simulink model "Discomfort"  (R2023b)
settings: Solver=VariableStepAuto  StartTime=0.0  StopTime=10  RelTol=1e-3
values from neighbouring files (symbols this model uses):
  a = 1.35    [Parameters.m]
  b = 1.5    [Parameters.m]
  d = 3    [Parameters.m]
  g = 9.81    [Parameters.m]
  I = 650    [Parameters.m]
  Kt = 14e4    (= 140000)    [Parameters.m]
  L = 3.7    [Parameters.m]
  Mw = 20    [Parameters.m]
  v = [1, 2, 3, 5, 8, 10]    [Parameters.m]
libraries: CarModelLibrary x9, simulink x6, SpeedBumpLibrary x4, spsRMSLib x3
settings Model: Creator=fb552  LastModifiedBy=Francesco
settings SolverCC: AlgebraicLoopSolver=TrustRegion
settings DataIOCC: ReturnWorkspaceOutputsName=SDOSimTest_Log
settings DebuggingCC: UnconnectedInputMsg=warning  UnconnectedOutputMsg=warning  UnconnectedLineMsg=warning
settings ModelReferenceCC: EnableRefExpFcnMdlSchedulingChecks=on

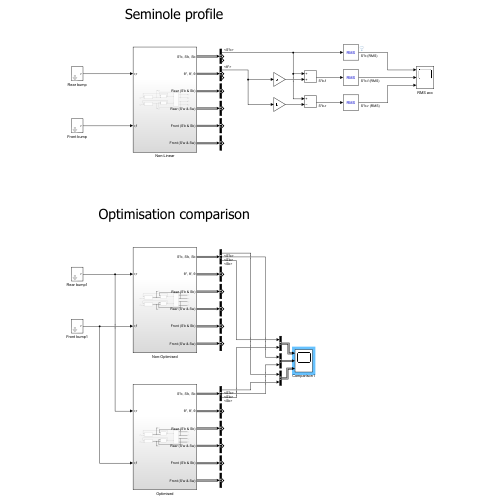
[thumbnail: Simulink's stored preview of the top-level diagram]
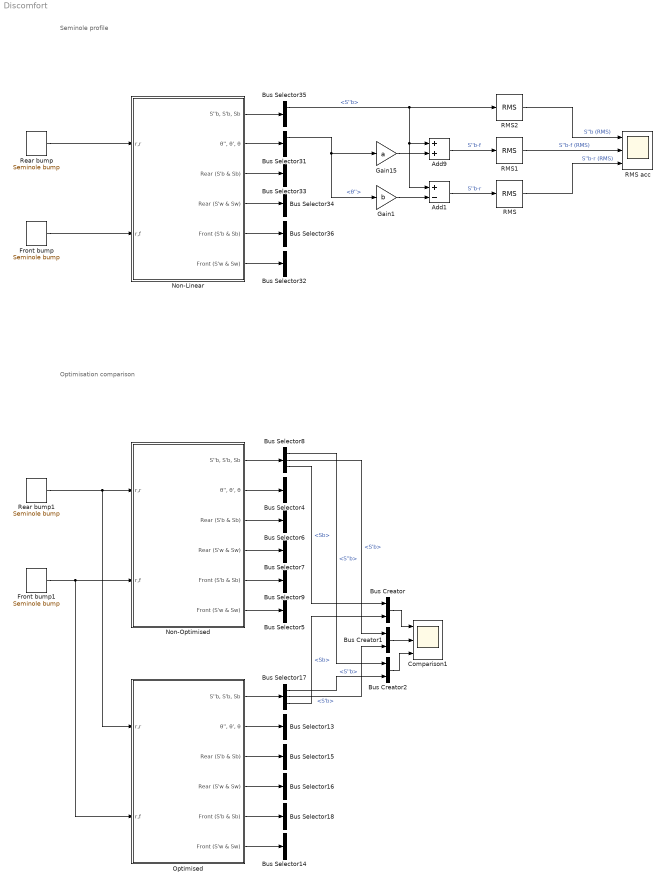
== system Discomfort ==
  note: Seminole profile
  note: Optimisation comparison
  Add1 : Sum  Inputs=+-
  Add9 : Sum
  Bus Creator : BusCreator  Inputs=2
  Bus Creator1 : BusCreator  Inputs=2
  Bus Creator2 : BusCreator  Inputs=2
  Bus Selector13 : BusSelector  OutputSignals=θ
  Bus Selector{5,7,14,16,32,34} (6 alike) : BusSelector  OutputSignals=Sw
  Bus Selector{6,9,15,18,33,36} (6 alike) : BusSelector  OutputSignals=Sb
  Bus Selector17 : BusSelector  OutputSignals=S''b,S'b,Sb
  Bus Selector31 : BusSelector  OutputSignals=θ'',θ',θ
  Bus Selector35 : BusSelector  OutputSignals=S''b,S'b,Sb
  Bus Selector4 : BusSelector  OutputSignals=θ
  Bus Selector8 : BusSelector  OutputSignals=S''b,S'b,Sb
  Comparison1 : Scope  NumInputPorts=3
  Front bump : SpeedBumpLibrary/Seminole bump  h=h  d=d  L=L+d  v=v(5)  delta=0  n=5
  Front bump1 : SpeedBumpLibrary/Seminole bump  h=h  d=d  L=L+d  v=v(5)  delta=0  n=5
  Gain1 : Gain  Gain=b
  Gain15 : Gain  Gain=a
  Non-Linear : Subsystem
  Non-Optimised : Subsystem
  Optimised : Subsystem
  RMS : spsRMSLib/RMS  TrueRMS=on  Freq=60  RMSInit=120  Ts=0
  RMS acc : Scope  NumInputPorts=3
  RMS1 : spsRMSLib/RMS  TrueRMS=on  Freq=60  RMSInit=120  Ts=0
  RMS2 : spsRMSLib/RMS  TrueRMS=on  Freq=60  RMSInit=120  Ts=0
  Rear bump : SpeedBumpLibrary/Seminole bump  h=h  d=d  L=L+d  v=v(5)  delta=a+b  n=5
  Rear bump1 : SpeedBumpLibrary/Seminole bump  h=h  d=d  L=L+d  v=v(5)  delta=a+b  n=5
  wires:
  Non-Linear/2("θ'', θ', θ") -> Bus Selector31/1
  Non-Linear/6(Front (S'w & Sw)) -> Bus Selector32/1
  Non-Linear/4(Rear (S'w & Sw)) -> Bus Selector34/1
  Non-Linear/5(Front (S'b & Sb)) -> Bus Selector36/1
  Non-Linear/1("S''b, S'b, Sb") -> Bus Selector35/1
  Non-Linear/3(Rear (S'b & Sb)) -> Bus Selector33/1
  Gain15/1 -> Add9/2
  Gain1/1 -> Add1/2
  Bus Selector35/1 -> Add1/1, Add9/1, RMS2/1  "<S''b>"
  Bus Selector31/1 -> Gain1/1, Gain15/1  "<θ''>"
  Add1/1 -> RMS/1  "S''b-r"
  Add9/1 -> RMS1/1  "S''b-f"
  RMS1/1 -> RMS acc/2  "S''b-f (RMS)"
  RMS2/1 -> RMS acc/1  "S''b (RMS)"
  RMS/1 -> RMS acc/3  "S''b-r (RMS)"
  Non-Optimised/1("S''b, S'b, Sb") -> Bus Selector8/1
  Non-Optimised/3(Rear (S'b & Sb)) -> Bus Selector6/1
  Non-Optimised/5(Front (S'b & Sb)) -> Bus Selector9/1
  Non-Optimised/2("θ'', θ', θ") -> Bus Selector4/1
  Non-Optimised/4(Rear (S'w & Sw)) -> Bus Selector7/1
  Non-Optimised/6(Front (S'w & Sw)) -> Bus Selector5/1
  Optimised/6(Front (S'w & Sw)) -> Bus Selector14/1
  Optimised/4(Rear (S'w & Sw)) -> Bus Selector16/1
  Optimised/3(Rear (S'b & Sb)) -> Bus Selector15/1
  Optimised/5(Front (S'b & Sb)) -> Bus Selector18/1
  Optimised/2("θ'', θ', θ") -> Bus Selector13/1
  Front bump1/1 -> Optimised/2(r,f), Non-Optimised/2(r,f)
  Rear bump1/1 -> Optimised/1(r,r), Non-Optimised/1(r,r)
  Optimised/1("S''b, S'b, Sb") -> Bus Selector17/1
  Rear bump/1 -> Non-Linear/1(r,r)
  Front bump/1 -> Non-Linear/2(r,f)
  Bus Creator2/1 -> Comparison1/3
  Bus Creator1/1 -> Comparison1/2
  Bus Creator/1 -> Comparison1/1
  Bus Selector17/1 -> Bus Creator2/2  "<S''b>"
  Bus Selector8/1 -> Bus Creator2/1  "<S''b>"
  Bus Selector8/2 -> Bus Creator1/1  "<S'b>"
  Bus Selector17/2 -> Bus Creator1/2  "<S'b>"
  Bus Selector17/3 -> Bus Creator/2  "<Sb>"
  Bus Selector8/3 -> Bus Creator/1  "<Sb>"

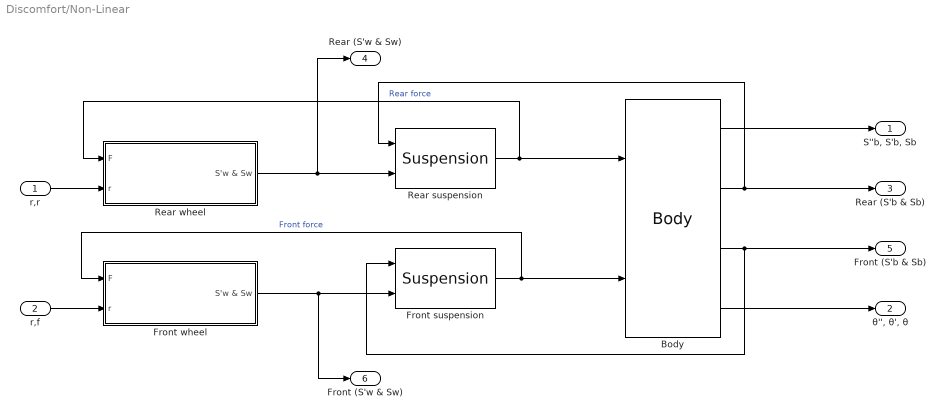
== system Discomfort/Non-Linear ==
  r,r : Inport
  r,f : Inport  Port=2
  Body : CarModelLibrary/Body  mb=Mb  I=I  a=a  b=b
  Front suspension : CarModelLibrary/Suspension  ks=Ks  ksstiff=Kstiff  x0=x0  csb=Csc  csr=Cse
  Front wheel : Subsystem  AncestorBlock=CarModelLibrary/Wheel  mask{mw=Mw, Kt=Kt, g=g}
      mask prompts: mw "Wheel Mass (Kg)"; Kt "Tyre Stiffness"; g "Gravitational acceleration"
  Rear suspension : CarModelLibrary/Suspension  ks=Ks  ksstiff=Kstiff  x0=x0  csb=Csc  csr=Cse
  Rear wheel : Subsystem  AncestorBlock=CarModelLibrary/Wheel  mask{mw=Mw, Kt=Kt, g=g}
      mask prompts: mw "Wheel Mass (Kg)"; Kt "Tyre Stiffness"; g "Gravitational acceleration"
  "S''b, S'b, Sb" : Outport
  "θ'', θ', θ" : Outport  Port=2
  Rear (S'b & Sb) : Outport  Port=3
  Rear (S'w & Sw) : Outport  Port=4
  Front (S'b & Sb) : Outport  Port=5
  Front (S'w & Sw) : Outport  Port=6
  wires:
  Body/1 -> "S''b, S'b, Sb"/1
  Body/2 -> Rear suspension/1, Rear (S'b & Sb)/1
  Front wheel/1(S'w & Sw) -> Front suspension/2, Front (S'w & Sw)/1
  Rear wheel/1(S'w & Sw) -> Rear suspension/2, Rear (S'w & Sw)/1
  Body/4 -> "θ'', θ', θ"/1
  Body/3 -> Front suspension/1, Front (S'b & Sb)/1
  Rear suspension/1 -> Body/1, Rear wheel/1(F)  "Rear force"
  r,r/1 -> Rear wheel/2(r)
  r,f/1 -> Front wheel/2(r)
  Front suspension/1 -> Front wheel/1(F), Body/2  "Front force"

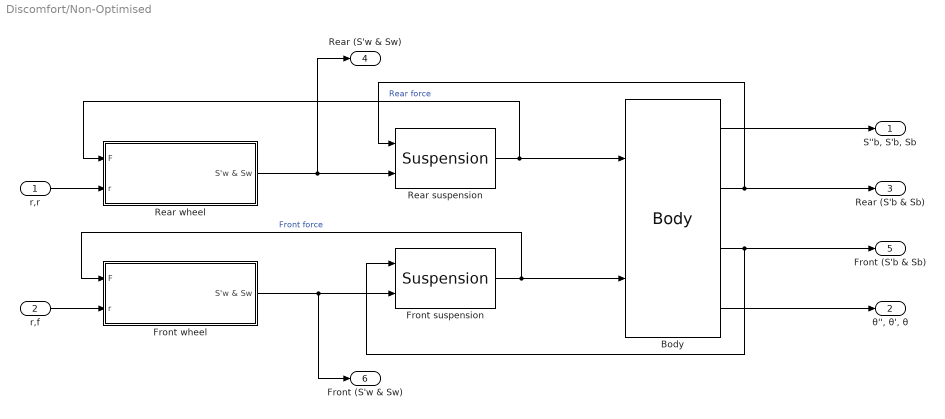
== system Discomfort/Non-Optimised ==
  r,r : Inport
  r,f : Inport  Port=2
  Body : CarModelLibrary/Body  mb=Mb  I=I  a=a  b=b
  Front suspension : CarModelLibrary/Suspension  ks=2e4  ksstiff=20  x0=x0  csb=600  csr=1200
  Front wheel : Subsystem  AncestorBlock=CarModelLibrary/Wheel  mask{mw=Mw, Kt=Kt, g=g}
      mask prompts: mw "Wheel Mass (Kg)"; Kt "Tyre Stiffness"; g "Gravitational acceleration"
  Rear suspension : CarModelLibrary/Suspension  ks=2e4  ksstiff=20  x0=x0  csb=600  csr=1200
  Rear wheel : Subsystem  AncestorBlock=CarModelLibrary/Wheel  mask{mw=Mw, Kt=Kt, g=g}
      mask prompts: mw "Wheel Mass (Kg)"; Kt "Tyre Stiffness"; g "Gravitational acceleration"
  "S''b, S'b, Sb" : Outport
  "θ'', θ', θ" : Outport  Port=2
  Rear (S'b & Sb) : Outport  Port=3
  Rear (S'w & Sw) : Outport  Port=4
  Front (S'b & Sb) : Outport  Port=5
  Front (S'w & Sw) : Outport  Port=6
  wires:
  Body/1 -> "S''b, S'b, Sb"/1
  Body/2 -> Rear suspension/1, Rear (S'b & Sb)/1
  Front wheel/1(S'w & Sw) -> Front suspension/2, Front (S'w & Sw)/1
  Rear wheel/1(S'w & Sw) -> Rear suspension/2, Rear (S'w & Sw)/1
  Body/4 -> "θ'', θ', θ"/1
  Body/3 -> Front suspension/1, Front (S'b & Sb)/1
  Rear suspension/1 -> Body/1, Rear wheel/1(F)  "Rear force"
  r,r/1 -> Rear wheel/2(r)
  r,f/1 -> Front wheel/2(r)
  Front suspension/1 -> Front wheel/1(F), Body/2  "Front force"

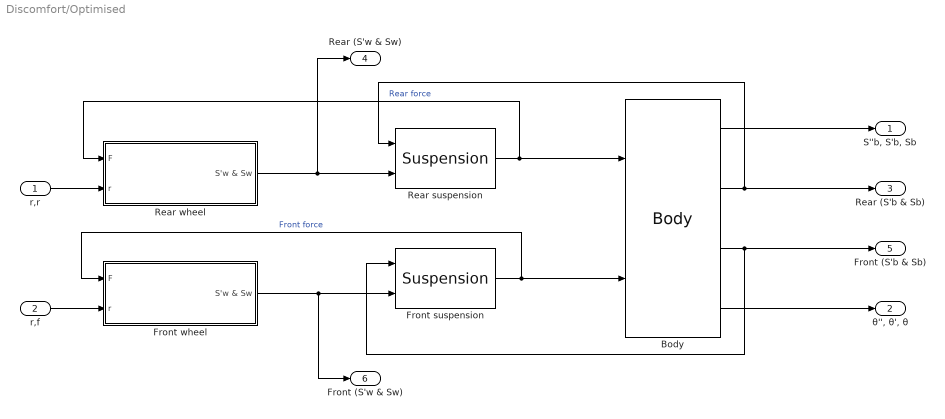
== system Discomfort/Optimised ==
  r,r : Inport
  r,f : Inport  Port=2
  Body : CarModelLibrary/Body  mb=Mb  I=I  a=a  b=b
  Front suspension : CarModelLibrary/Suspension  ks=Ks  ksstiff=Kstiff  x0=x0  csb=Csc  csr=Cse
  Front wheel : Subsystem  AncestorBlock=CarModelLibrary/Wheel  mask{mw=Mw, Kt=Kt, g=g}
      mask prompts: mw "Wheel Mass (Kg)"; Kt "Tyre Stiffness"; g "Gravitational acceleration"
  Rear suspension : CarModelLibrary/Suspension  ks=Ks  ksstiff=Kstiff  x0=x0  csb=Csc  csr=Cse
  Rear wheel : Subsystem  AncestorBlock=CarModelLibrary/Wheel  mask{mw=Mw, Kt=Kt, g=g}
      mask prompts: mw "Wheel Mass (Kg)"; Kt "Tyre Stiffness"; g "Gravitational acceleration"
  "S''b, S'b, Sb" : Outport
  "θ'', θ', θ" : Outport  Port=2
  Rear (S'b & Sb) : Outport  Port=3
  Rear (S'w & Sw) : Outport  Port=4
  Front (S'b & Sb) : Outport  Port=5
  Front (S'w & Sw) : Outport  Port=6
  wires:
  Body/1 -> "S''b, S'b, Sb"/1
  Body/2 -> Rear suspension/1, Rear (S'b & Sb)/1
  Front wheel/1(S'w & Sw) -> Front suspension/2, Front (S'w & Sw)/1
  Rear wheel/1(S'w & Sw) -> Rear suspension/2, Rear (S'w & Sw)/1
  Body/4 -> "θ'', θ', θ"/1
  Body/3 -> Front suspension/1, Front (S'b & Sb)/1
  Rear suspension/1 -> Body/1, Rear wheel/1(F)  "Rear force"
  r,r/1 -> Rear wheel/2(r)
  r,f/1 -> Front wheel/2(r)
  Front suspension/1 -> Front wheel/1(F), Body/2  "Front force"

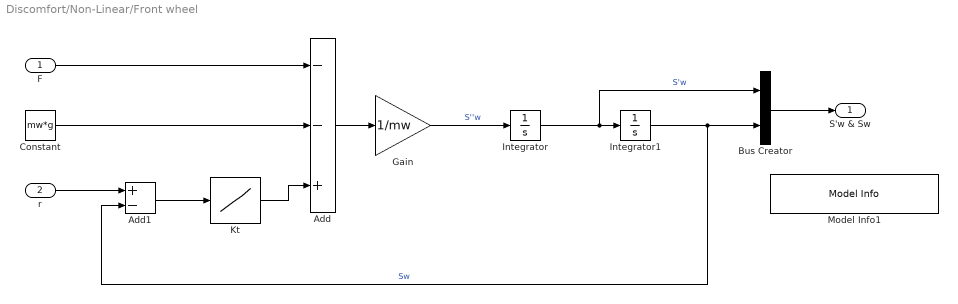
== system Discomfort/Non-Linear/Front wheel ==
  F : Inport
  r : Inport  Port=2
  Add : Sum  Inputs=--+
  Add1 : Sum  Inputs=+-
  Bus Creator : BusCreator  Inputs=2
  Constant : Constant  Value=mw*g
  Gain : Gain  Gain=1/mw
  Integrator : Integrator
  Integrator1 : Integrator
  Kt : Lookup_n-D  NumberOfTableDimensions=1  BreakpointsForDimension1=[-1, 0, 1]  Table=[0, 0, Kt]  InternalRulePriority=Speed  RndMeth=Simplest
  Model Info1 : simulink/Model-Wide Utilities/Model Info  Frame=on  DisplayStringWithTags=m * S''w = -F + Kt (r-S) - m*g  HorizontalTextAlignment=Center  LeftAlignmentValue=0.5
  S'w & Sw : Outport
  wires:
  Kt/1 -> Add/3
  F/1 -> Add/1
  Constant/1 -> Add/2
  Gain/1 -> Integrator/1  "S''w"
  Add/1 -> Gain/1
  Integrator1/1 -> Add1/2, Bus Creator/2  "Sw"
  Bus Creator/1 -> S'w & Sw/1
  Integrator/1 -> Integrator1/1, Bus Creator/1  "S'w"
  Add1/1 -> Kt/1
  r/1 -> Add1/1

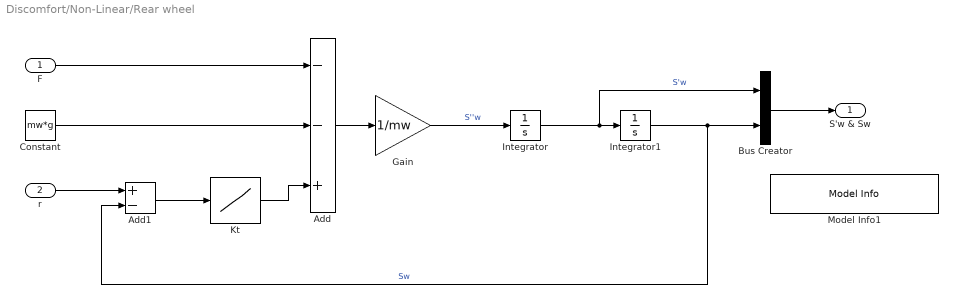
== system Discomfort/Non-Linear/Rear wheel ==
  F : Inport
  r : Inport  Port=2
  Add : Sum  Inputs=--+
  Add1 : Sum  Inputs=+-
  Bus Creator : BusCreator  Inputs=2
  Constant : Constant  Value=mw*g
  Gain : Gain  Gain=1/mw
  Integrator : Integrator
  Integrator1 : Integrator
  Kt : Lookup_n-D  NumberOfTableDimensions=1  BreakpointsForDimension1=[-1, 0, 1]  Table=[0, 0, Kt]  InternalRulePriority=Speed  RndMeth=Simplest
  Model Info1 : simulink/Model-Wide Utilities/Model Info  Frame=on  DisplayStringWithTags=m * S''w = -F + Kt (r-S) - m*g  HorizontalTextAlignment=Center  LeftAlignmentValue=0.5
  S'w & Sw : Outport
  wires:
  Kt/1 -> Add/3
  F/1 -> Add/1
  Constant/1 -> Add/2
  Gain/1 -> Integrator/1  "S''w"
  Add/1 -> Gain/1
  Integrator1/1 -> Add1/2, Bus Creator/2  "Sw"
  Bus Creator/1 -> S'w & Sw/1
  Integrator/1 -> Integrator1/1, Bus Creator/1  "S'w"
  Add1/1 -> Kt/1
  r/1 -> Add1/1

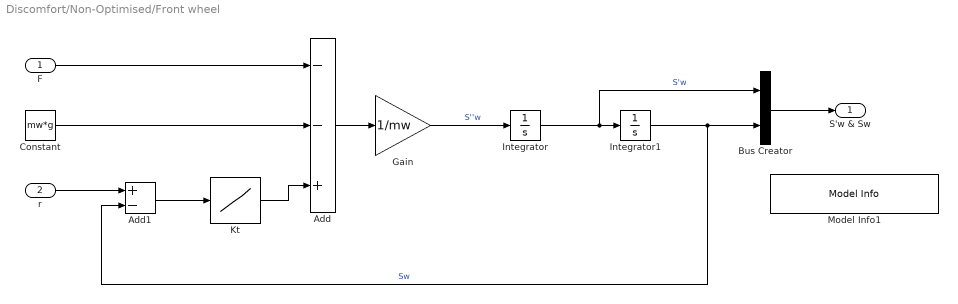
== system Discomfort/Non-Optimised/Front wheel ==
  F : Inport
  r : Inport  Port=2
  Add : Sum  Inputs=--+
  Add1 : Sum  Inputs=+-
  Bus Creator : BusCreator  Inputs=2
  Constant : Constant  Value=mw*g
  Gain : Gain  Gain=1/mw
  Integrator : Integrator
  Integrator1 : Integrator
  Kt : Lookup_n-D  NumberOfTableDimensions=1  BreakpointsForDimension1=[-1, 0, 1]  Table=[0, 0, Kt]  InternalRulePriority=Speed  RndMeth=Simplest
  Model Info1 : simulink/Model-Wide Utilities/Model Info  Frame=on  DisplayStringWithTags=m * S''w = -F + Kt (r-S) - m*g  HorizontalTextAlignment=Center  LeftAlignmentValue=0.5
  S'w & Sw : Outport
  wires:
  Kt/1 -> Add/3
  F/1 -> Add/1
  Constant/1 -> Add/2
  Gain/1 -> Integrator/1  "S''w"
  Add/1 -> Gain/1
  Integrator1/1 -> Add1/2, Bus Creator/2  "Sw"
  Bus Creator/1 -> S'w & Sw/1
  Integrator/1 -> Integrator1/1, Bus Creator/1  "S'w"
  Add1/1 -> Kt/1
  r/1 -> Add1/1

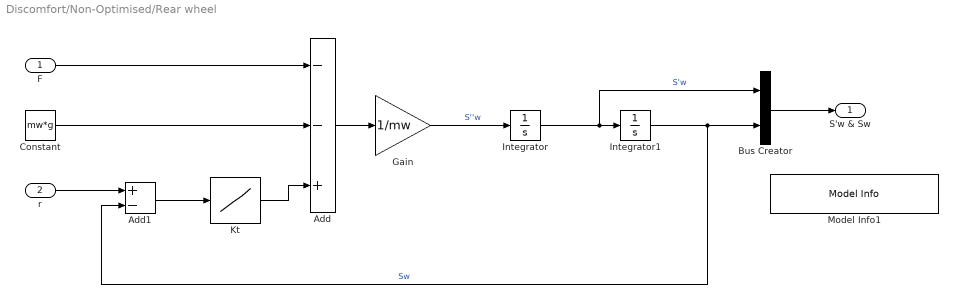
== system Discomfort/Non-Optimised/Rear wheel ==
  F : Inport
  r : Inport  Port=2
  Add : Sum  Inputs=--+
  Add1 : Sum  Inputs=+-
  Bus Creator : BusCreator  Inputs=2
  Constant : Constant  Value=mw*g
  Gain : Gain  Gain=1/mw
  Integrator : Integrator
  Integrator1 : Integrator
  Kt : Lookup_n-D  NumberOfTableDimensions=1  BreakpointsForDimension1=[-1, 0, 1]  Table=[0, 0, Kt]  InternalRulePriority=Speed  RndMeth=Simplest
  Model Info1 : simulink/Model-Wide Utilities/Model Info  Frame=on  DisplayStringWithTags=m * S''w = -F + Kt (r-S) - m*g  HorizontalTextAlignment=Center  LeftAlignmentValue=0.5
  S'w & Sw : Outport
  wires:
  Kt/1 -> Add/3
  F/1 -> Add/1
  Constant/1 -> Add/2
  Gain/1 -> Integrator/1  "S''w"
  Add/1 -> Gain/1
  Integrator1/1 -> Add1/2, Bus Creator/2  "Sw"
  Bus Creator/1 -> S'w & Sw/1
  Integrator/1 -> Integrator1/1, Bus Creator/1  "S'w"
  Add1/1 -> Kt/1
  r/1 -> Add1/1

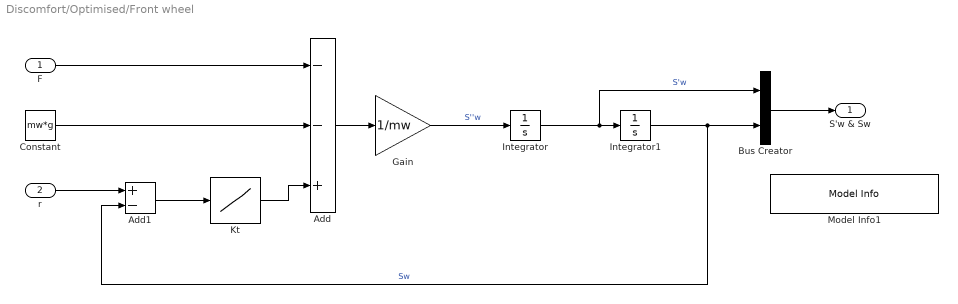
== system Discomfort/Optimised/Front wheel ==
  F : Inport
  r : Inport  Port=2
  Add : Sum  Inputs=--+
  Add1 : Sum  Inputs=+-
  Bus Creator : BusCreator  Inputs=2
  Constant : Constant  Value=mw*g
  Gain : Gain  Gain=1/mw
  Integrator : Integrator
  Integrator1 : Integrator
  Kt : Lookup_n-D  NumberOfTableDimensions=1  BreakpointsForDimension1=[-1, 0, 1]  Table=[0, 0, Kt]  InternalRulePriority=Speed  RndMeth=Simplest
  Model Info1 : simulink/Model-Wide Utilities/Model Info  Frame=on  DisplayStringWithTags=m * S''w = -F + Kt (r-S) - m*g  HorizontalTextAlignment=Center  LeftAlignmentValue=0.5
  S'w & Sw : Outport
  wires:
  Kt/1 -> Add/3
  F/1 -> Add/1
  Constant/1 -> Add/2
  Gain/1 -> Integrator/1  "S''w"
  Add/1 -> Gain/1
  Integrator1/1 -> Add1/2, Bus Creator/2  "Sw"
  Bus Creator/1 -> S'w & Sw/1
  Integrator/1 -> Integrator1/1, Bus Creator/1  "S'w"
  Add1/1 -> Kt/1
  r/1 -> Add1/1

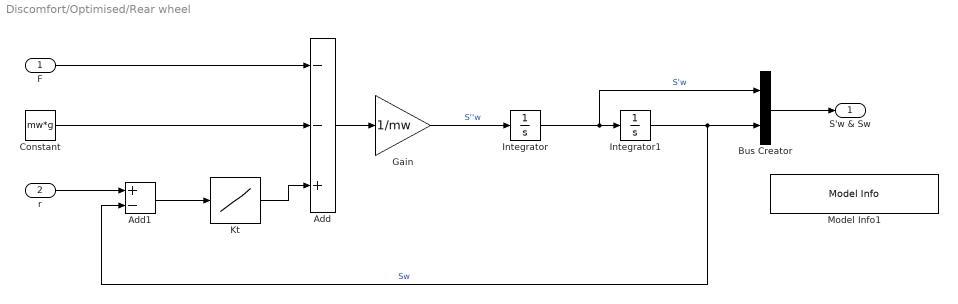
== system Discomfort/Optimised/Rear wheel ==
  F : Inport
  r : Inport  Port=2
  Add : Sum  Inputs=--+
  Add1 : Sum  Inputs=+-
  Bus Creator : BusCreator  Inputs=2
  Constant : Constant  Value=mw*g
  Gain : Gain  Gain=1/mw
  Integrator : Integrator
  Integrator1 : Integrator
  Kt : Lookup_n-D  NumberOfTableDimensions=1  BreakpointsForDimension1=[-1, 0, 1]  Table=[0, 0, Kt]  InternalRulePriority=Speed  RndMeth=Simplest
  Model Info1 : simulink/Model-Wide Utilities/Model Info  Frame=on  DisplayStringWithTags=m * S''w = -F + Kt (r-S) - m*g  HorizontalTextAlignment=Center  LeftAlignmentValue=0.5
  S'w & Sw : Outport
  wires:
  Kt/1 -> Add/3
  F/1 -> Add/1
  Constant/1 -> Add/2
  Gain/1 -> Integrator/1  "S''w"
  Add/1 -> Gain/1
  Integrator1/1 -> Add1/2, Bus Creator/2  "Sw"
  Bus Creator/1 -> S'w & Sw/1
  Integrator/1 -> Integrator1/1, Bus Creator/1  "S'w"
  Add1/1 -> Kt/1
  r/1 -> Add1/1
